simulink model "controller"  (R2023a)
settings: Solver=VariableStepAuto  StartTime=0.0  StopTime=10.0  RelTol=1e-3
undefined symbols (not defined in the file): DiscIntNeverNeededParam
libraries: simulink x1
settings Model: Creator=pengda  LastModifiedBy=pengda

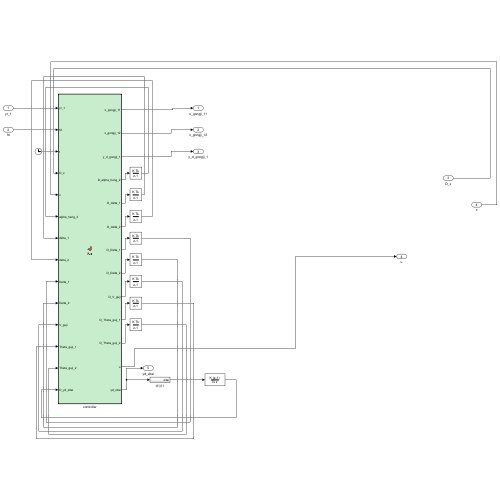
[thumbnail: Simulink's stored preview of the top-level diagram]
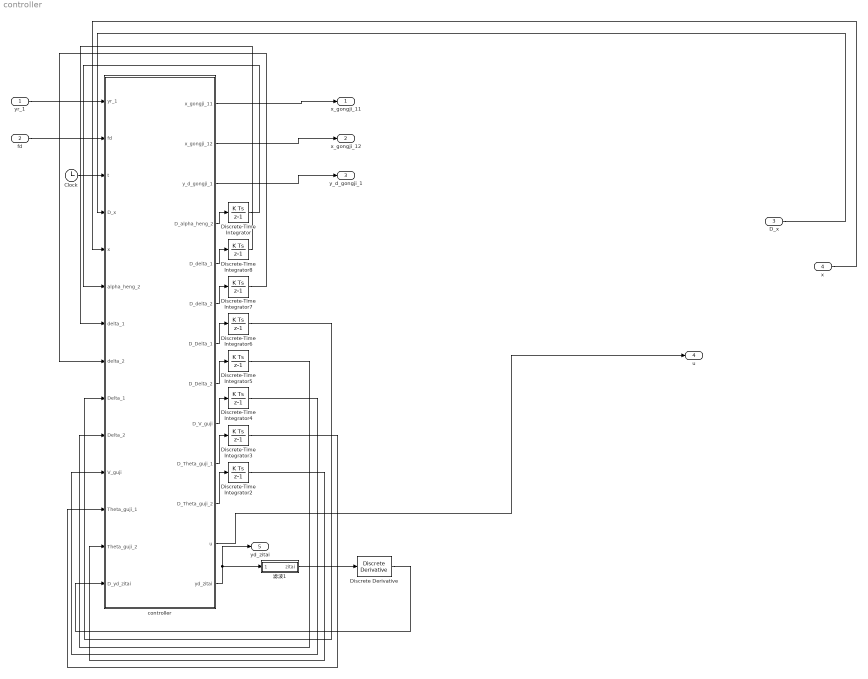
== system controller ==
  yr_1 : Inport
  fd : Inport  Port=2
  D_x : Inport  Port=3
  x : Inport  Port=4
  Clock : Clock
  Discrete Derivative : simulink/Discrete/Discrete Derivative  gainval=1.0  ICPrevScaledInput=0.0  OutMin=[]  OutMax=[]  OutDataType=fixdt(1, 16)  OutScaling=2^-10  DoSatur=off
  Discrete-Time Integrator{,5..8} (5 alike) : DiscreteIntegrator  InitialCondition=[0;0;0;0;0;0]  SampleTime=-1  ICPrevOutput=DiscIntNeverNeededParam  ICPrevScaledInput=DiscIntNeverNeededParam
  Discrete-Time Integrator2 : DiscreteIntegrator  InitialCondition=[1.2;1.2;1.2;0.2;0.2;0.2]  SampleTime=-1  ICPrevOutput=DiscIntNeverNeededParam  ICPrevScaledInput=DiscIntNeverNeededParam
  Discrete-Time Integrator3 : DiscreteIntegrator  InitialCondition=[2.2;2.2;2.2;0;0;0]  SampleTime=-1  ICPrevOutput=DiscIntNeverNeededParam  ICPrevScaledInput=DiscIntNeverNeededParam
  Discrete-Time Integrator4 : DiscreteIntegrator  InitialCondition=[4;4;4;0;0;0]  SampleTime=-1  ICPrevOutput=DiscIntNeverNeededParam  ICPrevScaledInput=DiscIntNeverNeededParam
  controller : MATLAB Function  TreatAsAtomicUnit=on
  滤波1 : Subsystem
  x_gongji_11 : Outport
  x_gongji_12 : Outport  Port=2
  y_d_gongji_1 : Outport  Port=3
  u : Outport  Port=4
  yd_zitai : Outport  Port=5
  wires:
  controller/8(D_Delta_2) -> Discrete-Time Integrator5/1
  controller/1(x_gongji_11) -> x_gongji_11/1
  controller/12(u) -> u/1
  controller/3(y_d_gongji_1) -> y_d_gongji_1/1
  controller/4(D_alpha_heng_2) -> Discrete-Time Integrator/1
  controller/13(yd_zitai) -> yd_zitai/1, 滤波1/1(" ")
  controller/10(D_Theta_guji_1) -> Discrete-Time Integrator3/1
  controller/11(D_Theta_guji_2) -> Discrete-Time Integrator2/1
  滤波1/1(zitai) -> Discrete Derivative/1
  D_x/1 -> controller/4(D_x)
  Discrete-Time Integrator3/1 -> controller/12(Theta_guji_1)
  fd/1 -> controller/2(fd)
  Clock/1 -> controller/3(t)
  controller/5(D_delta_1) -> Discrete-Time Integrator8/1
  yr_1/1 -> controller/1(yr_1)
  Discrete Derivative/1 -> controller/14(D_yd_zitai)
  controller/2(x_gongji_12) -> x_gongji_12/1
  Discrete-Time Integrator8/1 -> controller/7(delta_1)
  Discrete-Time Integrator6/1 -> controller/9(Delta_1)
  controller/6(D_delta_2) -> Discrete-Time Integrator7/1
  Discrete-Time Integrator5/1 -> controller/10(Delta_2)
  controller/9(D_V_guji) -> Discrete-Time Integrator4/1
  Discrete-Time Integrator2/1 -> controller/13(Theta_guji_2)
  Discrete-Time Integrator/1 -> controller/6(alpha_heng_2)
  controller/7(D_Delta_1) -> Discrete-Time Integrator6/1
  Discrete-Time Integrator4/1 -> controller/11(V_guji)
  Discrete-Time Integrator7/1 -> controller/8(delta_2)
  x/1 -> controller/5(x)

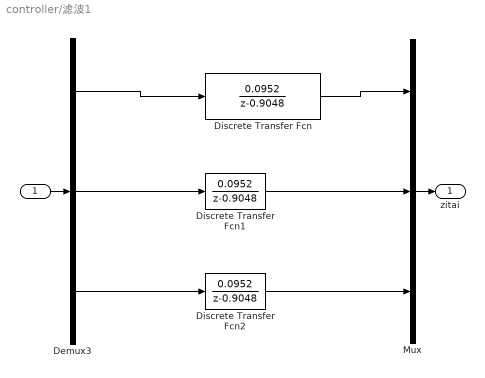
== system controller/滤波1 ==
  " " : Inport
  Demux3 : Demux  Outputs=3
  Discrete Transfer Fcn : DiscreteTransferFcn  Numerator=[0.0952]  Denominator=[1, -0.9048]
  Discrete Transfer Fcn1 : DiscreteTransferFcn  Numerator=[0.0952]  Denominator=[1, -0.9048]
  Discrete Transfer Fcn2 : DiscreteTransferFcn  Numerator=[0.0952]  Denominator=[1, -0.9048]
  Mux : Mux  Inputs=3
  zitai : Outport  VectorParamsAs1DForOutWhenUnconnected=off
  wires:
  Demux3/3 -> Discrete Transfer Fcn2/1
  Discrete Transfer Fcn2/1 -> Mux/3
  Discrete Transfer Fcn/1 -> Mux/1
  Discrete Transfer Fcn1/1 -> Mux/2
  Demux3/1 -> Discrete Transfer Fcn/1
  Demux3/2 -> Discrete Transfer Fcn1/1
  Mux/1 -> zitai/1
  " "/1 -> Demux3/1

== matlab function controller/controller ==
  data: yr_1 input; fd input; t input; D_x input; x input; x_gongji_11 output; x_gongji_12 output; y_d_gongji_1 output; alpha_heng_2 input; delta_1 input; delta_2 input; Delta_1 input; Delta_2 input; V_guji input; Theta_guji_1 input; Theta_guji_2 input; D_alpha_heng_2 output; D_delta_1 output; D_delta_2 output; D_Delta_1 output; D_Delta_2 output; D_V_guji output; D_Theta_guji_1 output; D_Theta_guji_2 output; u output; D_yd_zitai input; yd_zitai output
function [x_gongji_11,x_gongji_12,y_d_gongji_1, D_alpha_heng_2, D_delta_1, D_delta_2, D_Delta_1,D_Delta_2, D_V_guji, D_Theta_guji_1,D_Theta_guji_2, u, yd_zitai]  =   fcn( yr_1, fd, t, D_x, x, alpha_heng_2, delta_1,delta_2, Delta_1,Delta_2, V_guji, Theta_guji_1,Theta_guji_2,D_yd_zitai)
%%
%%%%%%%%%%%%%%%%%%%%%%%%%%%%%%%%%%%%%%%%%%%%%%%%%%%%%%%%%%%%%%%%%%%%%%%%%%%%%%%%%%%%%%%%%%%%%%%%%%%%%%%%%%%%%%%%%%%%%%%%%%%%%
%                                      控制器参数
% % 通信拓步图参数
%   X          Y
 af1 = 1;    %领航者
 af2 = 0;    %2号
 af3 = 0;    %3号
 af4 = 0;    %4号
 af5 = 0;    %5号

%%%%%%%%%%%%%%%%%%%%%%%%%%%%
%%%%%%%%%%%%%%%%%%%%%%%%%
%%
%动力学参数
m = 1.8;
g = 9.81;

fx=0.001;%平移阻力系数
fy=0.001;
fz=0.001;
f_theta=0.15;
f_phi=0.15;
f_psi=0.15;

I_xx = 0.75;      % 四旋翼x轴转动惯量(kg·m^2)
I_yy = 0.75;      % 四旋翼y轴转动惯量(kg·m^2)
I_zz = 1.5;       % 四旋翼z轴转动惯量(kg·m^2)
J_RP = 0.0000616;   % 整个电机转子和螺旋桨绕转轴的总转动惯量(kg·m^2)
d = 0.2;          % 机体中心和任一电机的距离(m)


%执行器故障
rho_1 = 0.8;
rho_2 = 0.8;
rho_3 = 1;
rho_4 = 1;
rho_5 = 1;
rho_6 = 1;

yita_1 = 0.02*cos(0.2*t);
yita_2 = 0.02*cos(0.2*t);
yita_3 = 0;
yita_4 = 0;
yita_5 = 0;
yita_6 = 0;

%滤波器参数  重要<1
epsilon_12=0.01;
epsilon_22=0.01;
epsilon_32=0.01;
epsilon_42=0.03;
epsilon_52=0.05;
epsilon_62=0.08;

%控制器参数
T=3;
zeta=1;

c=70;
l=0.03;%0.03

t_1=12;
t_2=11;
t_3=11;
t_4=2;
t_5=2;
t_6=2;

k_11=60;%重要
k_21=40;
k_31=50;
k_41=40;
k_51=40;
k_61=40;

k_12=60;%重要
k_22=40;
k_32=50;
k_42=40;
k_52=40;
k_62=40;

l_11=1.5;
l_21=1.5;
l_31=1.5;
l_41=1.5;
l_51=1.5;
l_61=1.5;

l_12=1;
l_22=1;
l_32=1;
l_42=1;
l_52=1;
l_62=1;

sigma_11=32;
sigma_21=48;
sigma_31=45;
sigma_41=32;
sigma_51=37;
sigma_61=36;

sigma_12=3.6;%重要
sigma_22=3.5;
sigma_32=3.2;
sigma_42=2.7;
sigma_52=2.8;
sigma_62=3.1;

%
p=2;

E=10;

g_1=8;%重要
g_2=8;
g_3=8;
g_4=10;
g_5=10;
g_6=10;



%
D_X=D_x(1);
D_Y=D_x(2);
D_Z=D_x(3);
D_theta=D_x(4);
D_phi=D_x(5);
D_psi=D_x(6);

X=x(1);
Y=x(2);
Z=x(3);
theta=x(4);
phi=x(5);
psi=x(6);

yd_1=yr_1(1);
yd_2=yr_1(2);
yd_3=yr_1(3);

fd_1=fd(1);
fd_2=fd(2);
fd_3=fd(3);

fd_4=D_yd_zitai(1);
fd_5=D_yd_zitai(2);
fd_6=D_yd_zitai(3);

alpha_heng_12=alpha_heng_2(1);
alpha_heng_22=alpha_heng_2(2);
alpha_heng_32=alpha_heng_2(3);
alpha_heng_42=alpha_heng_2(4);
alpha_heng_52=alpha_heng_2(5);
alpha_heng_62=alpha_heng_2(6);

delta_11=delta_1(1);
delta_21=delta_1(2);
delta_31=delta_1(3);
delta_41=delta_1(4);
delta_51=delta_1(5);
delta_61=delta_1(6);

delta_12=delta_2(1);
delta_22=delta_2(2);
delta_32=delta_2(3);
delta_42=delta_2(4);
delta_52=delta_2(5);
delta_62=delta_2(6);

Delta_11=Delta_1(1);
Delta_21=Delta_1(2);
Delta_31=Delta_1(3);
Delta_41=Delta_1(4);
Delta_51=Delta_1(5);
Delta_61=Delta_1(6);

Delta_12=Delta_2(1);
Delta_22=Delta_2(2);
Delta_32=Delta_2(3);
Delta_42=Delta_2(4);
Delta_52=Delta_2(5);
Delta_62=Delta_2(6);

V_guji_1=V_guji(1);
V_guji_2=V_guji(2);
V_guji_3=V_guji(3);
V_guji_4=V_guji(4);
V_guji_5=V_guji(5);
V_guji_6=V_guji(6);

Theta_guji_11=Theta_guji_1(1);
Theta_guji_21=Theta_guji_1(2);
Theta_guji_31=Theta_guji_1(3);
Theta_guji_41=Theta_guji_1(4);
Theta_guji_51=Theta_guji_1(5);
Theta_guji_61=Theta_guji_1(6);

Theta_guji_12=Theta_guji_2(1);
Theta_guji_22=Theta_guji_2(2);
Theta_guji_32=Theta_guji_2(3);
Theta_guji_42=Theta_guji_2(4);
Theta_guji_52=Theta_guji_2(5);
Theta_guji_62=Theta_guji_2(6);


%%%%%%%%%%%%%%%%%%%%%%%%%%%%%%%%%%%%%%%%%%%%%%%%%%%%%%%%%%%%%%%%%%%%%%%%%%%%%%%%%%%%%%%%%%%%%%%%%%%%%%%%%%% 编队
%%%%%%%%%%%%%%%%%%%%%%%%%%%%%%%%%%%%%%%%%%%%%%%%%%%%%%%%%%%%%%%%%%%%%%%%%%%%%%%%%%%%%%%%%%%%%%%%%%%%%%%%%%%
%% 偏移量
% 偏差
y_offest_1 = -1;
y_offest_2 = -1;
y_offest_3 = 0;

x_offest_112 = 0;%对y_offest_1求导
x_offest_122 = 0;
x_offest_132 = 0;


% 编队信息
y_d_1 = yd_1 + y_offest_1;
y_d_2 = yd_2 + y_offest_2;
y_d_3 = yd_3 + y_offest_3;

%%%%%%%%%%%%%%%%%%%%%%%%%%%%%%%%%%%%%%%%%%%%%%%%%%%%%%%%%%%%%%%%%%%%%%%%%%%%%%%%%%%%%%%%%%%%%%%%%%%%%%%%%%% 欺骗攻击 
%%%%%%%%%%%%%%%%%%%%%%%%%%%%%%%%%%%%%%%%%%%%%%%%%%%%%%%%%%%%%%%%%%%%%%%%%%%%%%%%%%%%%%%%%%%%%%%%%%%%%%%%%%%
%% 欺骗攻击

if t<10
    o = 0;
else
    o = -0.01*cos(0.25*t);%更改后导数D_lambda更改
end

% o_1 = -0.2*cos(0.25*t);o_2 = -0.2*cos(0.25*t);o_3 = -0.2*cos(0.25*t);
% o_4 = -0.2*cos(0.25*t);o_5 = -0.2*cos(0.25*t);o_6 = -0.2*cos(0.25*t);

lambda = 1 + o;

if t<10
    D_lambda = 0; 
else
    D_lambda = 0.01*0.25*sin(0.25*t); 
end


% 实际状态一阶
x_gongji_111 = lambda * X ;
x_gongji_121 = lambda * Y ;
x_gongji_131 = lambda * Z ;
x_gongji_141 = lambda * theta ;
x_gongji_151 = lambda * phi ;
x_gongji_161 = lambda * psi ;

% 实际状态二阶
x_gongji_112 = lambda * D_X ;
x_gongji_122 = lambda * D_Y ;
x_gongji_132 = lambda * D_Z ;
x_gongji_142 = lambda * D_theta ;
x_gongji_152 = lambda * D_phi ;
x_gongji_162 = lambda * D_psi ;

% 期望状态
yd_gongji_1 = lambda * yd_1 ;
yd_gongji_2 = lambda * yd_2 ;
yd_gongji_3 = lambda * yd_3 ;


% 编队信息-攻击
y_d_gongji_11 = yd_gongji_1 + y_offest_1;
y_d_gongji_12 = yd_gongji_2 + y_offest_2;
y_d_gongji_13 = yd_gongji_3 + y_offest_3;


%%%%%%%%%%%%%%%%%%%%%%%%%%%%%%%%%%%%%%%%%%%%%%%%%%%%%%%%%%%%%%%%%%%%%%%%%%%%%%%%%%%%%%%%%%%%%%%%%%%%%%%%%%%  动力学模型 位置
%%%%%%%%%%%%%%%%%%%%%%%%%%%%%%%%%%%%%%%%%%%%%%%%%%%%%%%%%%%%%%%%%%%%%%%%%%%%%%%%%%%%%%%%%%%%%%%%%%%%%%%%%%%
%% 动力学模型  位置
%跟随者
F1=-fx*D_X/m ;
F2=-fy*D_Y/m ;
F3=-g-fz*D_Z/m ;

d_x=0.2*sin(t);d_y=0.0001*cos(t);d_z=0.15;
N1=d_x/m;
N2=d_y/m;
N3=d_z/m;

%%%%%%%%%%%%%%%%%%%%%%%%%%%%%%%%%%%%%%%%%%%%%%%%%%%%%%%%%%%%%%%%%%%%%%%%%%%%%%%%%%%%%%%%%%%%%%%%%%%%%%%%%%%  位置控制器
%%%%%%%%%%%%%%%%%%%%%%%%%%%%%%%%%%%%%%%%%%%%%%%%%%%%%%%%%%%%%%%%%%%%%%%%%%%%%%%%%%%%%%%%%%%%%%%%%%%%%%%%%%%
%% 一阶控制器

y_gongji_11 = x_gongji_111;  % y_gongji_i,m ; x_gongji_i,m,s
y_gongji_12 = x_gongji_121;
y_gongji_13 = x_gongji_131;

z_11 = 0 + g_1*(y_gongji_11-y_d_gongji_11);
z_21 = 0 + g_2*(y_gongji_12-y_d_gongji_12);
z_31 = 0 + g_3*(y_gongji_13-y_d_gongji_13);


if t >= 0 && t <= T 
    v = (1/((t+0.01)^2) - 1/(T^2))^(2*p) + zeta;  % eps是MATLAB内置极小值（~2.2e-16）
    D_v = -4*p * (1/((t+0.01)^2) - 1/(T^2))^(2*p - 1) / (t + 0.01)^3;
    % D_v=-(4*p/t^3)*(1/((t+0.01)^2) - 1/T^2)^(2*p-1);
else
    v = zeta;
    D_v = 0;
end


beta_1 = c*(v^2-z_11^2);    % beta_m 
beta_2 = c*(v^2-z_21^2); 
beta_3 = c*(v^2-z_31^2); 

if beta_1 > 0 && beta_1 <= l  
    h_1 = 1-(beta_1/l - 1)^(2*p);    % h_m 
elseif beta_1>l
    h_1=1;
else
    h_1=1;
end

if beta_2 > 0 && beta_2 <= l  
    h_2 = 1-(beta_2/l - 1)^(2*p);    % h_m 
elseif beta_2>l
    h_2=1;
else
    h_2=1;
end

if beta_3 > 0 && beta_3 <= l  
    h_3 = 1-(beta_3/l - 1)^(2*p);    % h_m 
elseif beta_3>l
    h_3=1;
else
    h_3=1;
end

H_11 = z_11/h_1;    % H_m,1
H_21 = z_21/h_2;
H_31 = z_31/h_3;


xi_11 = H_11;
xi_21 = H_21;
xi_31 = H_31;


if beta_1 > 0 && beta_1 <= l  
    mu_1 = 1/h_1 - (4*c*p/(l*h_1^2))*((beta_1/l - 1)^(2*p-1))*z_11^2;    % mu_m 
elseif beta_1>l
    mu_1=1;
else
    mu_1=1;
end

if beta_2 > 0 && beta_2 <= l  
    mu_2 = 1/h_2 - (4*c*p/(l*h_2^2))*((beta_2/l - 1)^(2*p-1))*z_21^2;    % mu_m 
elseif beta_2>l
    mu_2=1;
else
    mu_2=1;
end

if beta_3 > 0 && beta_3 <= l  
    mu_3 = 1/h_3 - (4*c*p/(l*h_3^2))*((beta_3/l - 1)^(2*p-1))*z_31^2;    % mu_m 
elseif beta_3>l
    mu_3=1;
else
    mu_3=1;
end

d_i= af2 + af3 + af4 + af5;

tau_1 = d_i + g_1;
tau_2 = d_i + g_2;
tau_3 = d_i + g_3;


B_1 = D_lambda*(lambda\tau_1)*x_gongji_111 - 0 - D_lambda*(lambda\g_1)*yd_gongji_1 - lambda*g_1*fd_1 - 0 + 0;
B_2 = D_lambda*(lambda\tau_2)*x_gongji_121 - 0 - D_lambda*(lambda\g_2)*yd_gongji_2 - lambda*g_2*fd_2 - 0 + 0;
B_3 = D_lambda*(lambda\tau_3)*x_gongji_131 - 0 - D_lambda*(lambda\g_3)*yd_gongji_3 - lambda*g_3*fd_3 - 0 + 0;




if beta_1 > 0 && beta_1 <= l  
    v_1 = (4*c*p/(l*h_1^2))*((beta_1/l - 1)^(2*p-1))*v*D_v*z_11;    % v_m 
elseif beta_1>l
    v_1=0;
else
    v_1=0;
end

if beta_2 > 0 && beta_2 <= l  
    v_2 = (4*c*p/(l*h_2^2))*((beta_2/l - 1)^(2*p-1))*v*D_v*z_21;    % v_m 
elseif beta_2>l
    v_2=0;
else
    v_2=0;
end

if beta_3 > 0 && beta_3 <= l  
    v_3 = (4*c*p/(l*h_3^2))*((beta_3/l - 1)^(2*p-1))*v*D_v*z_31;    % v_m 
elseif beta_3>l
    v_3=0;
else
    v_3=0;
end


alpha_11 = (-k_11*xi_11 - (Delta_11*mu_1^2*(E+1))/(4*sqrt(Delta_11^2*mu_1^2+sigma_11^2)) - Delta_11*mu_1^2*Theta_guji_11/sqrt(Delta_11^2*mu_1^2+sigma_11^2) - v_1 - (l_11*delta_11)/sqrt(delta_11^2+sigma_11^2))/(mu_1*tau_1);
alpha_21 = (-k_21*xi_21 - (Delta_21*mu_2^2*(E+1))/(4*sqrt(Delta_21^2*mu_2^2+sigma_21^2)) - Delta_21*mu_2^2*Theta_guji_21/sqrt(Delta_21^2*mu_2^2+sigma_21^2) - v_2 - (l_21*delta_21)/sqrt(delta_21^2+sigma_21^2))/(mu_2*tau_2);
alpha_31 = (-k_31*xi_31 - (Delta_31*mu_3^2*(E+1))/(4*sqrt(Delta_31^2*mu_3^2+sigma_31^2)) - Delta_31*mu_3^2*Theta_guji_31/sqrt(Delta_31^2*mu_3^2+sigma_31^2) - v_3 - (l_31*delta_31)/sqrt(delta_31^2+sigma_31^2))/(mu_3*tau_3);


D_Theta_guji_11 = Delta_11^2*mu_1^2/sqrt(Delta_11^2*mu_1^2+sigma_11^2) - sigma_11*Theta_guji_11;
D_Theta_guji_21 = Delta_21^2*mu_2^2/sqrt(Delta_21^2*mu_2^2+sigma_21^2) - sigma_21*Theta_guji_21;
D_Theta_guji_31 = Delta_31^2*mu_3^2/sqrt(Delta_31^2*mu_3^2+sigma_31^2) - sigma_31*Theta_guji_31;


D_delta_11 = -k_11*delta_11 + mu_1*tau_1*(alpha_heng_12-alpha_11) + mu_1*tau_1*delta_12 - (l_11*delta_11)/sqrt(delta_11^2+sigma_11^2);
D_delta_21 = -k_21*delta_21 + mu_2*tau_2*(alpha_heng_22-alpha_21) + mu_2*tau_2*delta_22 - (l_21*delta_21)/sqrt(delta_21^2+sigma_21^2);
D_delta_31 = -k_31*delta_31 + mu_3*tau_3*(alpha_heng_32-alpha_31) + mu_3*tau_3*delta_32 - (l_31*delta_31)/sqrt(delta_31^2+sigma_31^2);


D_Delta_11 = mu_1*tau_1*(Delta_12+alpha_11-x_offest_112) + mu_1*B_1 + v_1 + k_11*delta_11 + (l_11*delta_11)/sqrt(delta_11^2+sigma_11^2);
D_Delta_21 = mu_2*tau_2*(Delta_22+alpha_21-x_offest_122) + mu_2*B_2 + v_2 + k_21*delta_21 + (l_21*delta_21)/sqrt(delta_21^2+sigma_21^2);
D_Delta_31 = mu_3*tau_3*(Delta_32+alpha_31-x_offest_132) + mu_3*B_3 + v_3 + k_31*delta_31 + (l_31*delta_31)/sqrt(delta_31^2+sigma_31^2);



%% 二阶控制器


xi_12 = x_gongji_112-alpha_heng_12;
xi_22 = x_gongji_122-alpha_heng_22;
xi_32 = x_gongji_132-alpha_heng_32;


D_alpha_heng_12=(alpha_11-alpha_heng_12)/epsilon_12;
D_alpha_heng_22=(alpha_21-alpha_heng_22)/epsilon_22;
D_alpha_heng_32=(alpha_31-alpha_heng_32)/epsilon_32;


D_delta_12 = -k_12*delta_12 - (l_12*delta_12)/sqrt(delta_12^2+sigma_12^2);
D_delta_22 = -k_22*delta_22 - (l_22*delta_22)/sqrt(delta_22^2+sigma_22^2);
D_delta_32 = -k_32*delta_32 - (l_32*delta_32)/sqrt(delta_32^2+sigma_32^2);


D_Theta_guji_12 = Delta_12^2/sqrt(Delta_12^2+sigma_12^2) - sigma_12*Theta_guji_12;
D_Theta_guji_22 = Delta_22^2/sqrt(Delta_22^2+sigma_22^2) - sigma_22*Theta_guji_22;
D_Theta_guji_32 = Delta_32^2/sqrt(Delta_32^2+sigma_32^2) - sigma_32*Theta_guji_32;


pi_1 = k_12*xi_12 + (Delta_12*(E+1))/(4*sqrt(Delta_12^2+sigma_12^2)) + (Delta_12*Theta_guji_12)/sqrt(Delta_12^2+sigma_12^2) - D_alpha_heng_12 + (l_12*delta_12)/sqrt(delta_12^2+sigma_12^2) + Delta_11;
pi_2 = k_22*xi_22 + (Delta_22*(E+1))/(4*sqrt(Delta_22^2+sigma_22^2)) + (Delta_22*Theta_guji_22)/sqrt(Delta_22^2+sigma_22^2) - D_alpha_heng_22 + (l_22*delta_22)/sqrt(delta_22^2+sigma_22^2) + Delta_21;
pi_3 = k_32*xi_32 + (Delta_32*(E+1))/(4*sqrt(Delta_32^2+sigma_32^2)) + (Delta_32*Theta_guji_32)/sqrt(Delta_32^2+sigma_32^2) - D_alpha_heng_32 + (l_32*delta_32)/sqrt(delta_32^2+sigma_32^2) + Delta_31;


D_V_guji_1 = Delta_12*pi_1 - sigma_12*V_guji_1;
D_V_guji_2 = Delta_22*pi_2 - sigma_22*V_guji_2;
D_V_guji_3 = Delta_32*pi_3 - sigma_32*V_guji_3;


% u1 = -(Delta_12*V_guji_1^2*pi_1^2)/(C1*sqrt(Delta_12^2*V_guji_1^2*pi_1^2+t_1^2));
u1 = -(Delta_12*V_guji_1^2*pi_1^2)/(sqrt(Delta_12^2*V_guji_1^2*pi_1^2+t_1^2));
u2 = -(Delta_22*V_guji_2^2*pi_2^2)/(sqrt(Delta_22^2*V_guji_2^2*pi_2^2+t_2^2));
u3 = -(Delta_32*V_guji_3^2*pi_3^2)/(sqrt(Delta_32^2*V_guji_3^2*pi_3^2+t_3^2));


D_Delta_12 = D_lambda*(lambda\x_gongji_112) + lambda*rho_1*u1 - D_alpha_heng_12 + lambda*yita_1 + lambda*F1 + lambda*N1 + k_12*delta_12 + (l_12*delta_12)/sqrt(delta_12^2+sigma_12^2);
D_Delta_22 = D_lambda*(lambda\x_gongji_122) + lambda*rho_2*u2 - D_alpha_heng_22 + lambda*yita_2 + lambda*F2 + lambda*N2 + k_22*delta_22 + (l_22*delta_22)/sqrt(delta_22^2+sigma_22^2);
D_Delta_32 = D_lambda*(lambda\x_gongji_132) + lambda*rho_3*u3 - D_alpha_heng_32 + lambda*yita_3 + lambda*F3 + lambda*N3 + k_32*delta_32 + (l_32*delta_32)/sqrt(delta_32^2+sigma_32^2);


%%%%%%%%%%%%%%%%%%%%%%%%%%%%%%%%%%%%%%%%%%%%%%%%%%%%%%%%%%%%%%%%%%%%%%%%%%%%%%%%%%%%%%%%%%%%%%%%%%%%%%%%%%%  姿态动力学模型
%%%%%%%%%%%%%%%%%%%%%%%%%%%%%%%%%%%%%%%%%%%%%%%%%%%%%%%%%%%%%%%%%%%%%%%%%%%%%%%%%%%%%%%%%%%%%%%%%%%%%%%%%%%
%% 动力学模型
%跟随者 姿态
c_T = 120;    % 螺旋桨拉力系数
c_M = 0.033;  % 螺旋桨力矩系数
F = m *((u1)^2 + (u2)^2 + (u3)^2)^0.5;

w1= (abs(F/c_T + (2)^0.5*u1/(d*c_T) + (2)^0.5*u2/(d*c_T) + u3/(c_T*c_M))/4)^0.5;
w2= (abs(F/c_T - (2)^0.5*u1/(d*c_T) + (2)^0.5*u2/(d*c_T) - u3/(c_T*c_M))/4)^0.5;
w3= (abs(F/c_T - (2)^0.5*u1/(d*c_T) - (2)^0.5*u2/(d*c_T) + u3/(c_T*c_M))/4)^0.5;
w4= (abs(F/c_T + (2)^0.5*u1/(d*c_T) - (2)^0.5*u2/(d*c_T) - u3/(c_T*c_M))/4)^0.5;

Omega=-w1+w2-w3+w4;

a1=(I_zz-I_xx)/I_yy; a2=J_RP/I_yy; a3=f_theta/I_yy;
a4=(I_yy-I_zz)/I_xx; a5=J_RP/I_xx; a6=f_phi/I_xx;
a7=(I_xx-I_yy)/I_zz;a8=f_psi/I_zz;

F4=a1*D_phi*D_psi-a2*D_phi*Omega-a3*D_theta;
F5=a4*D_theta*D_psi-a5*D_theta*Omega-a6*D_phi;
F6=a7*D_theta*D_phi-a8*D_psi;

% d_x=0.2*sin(t);d_y=0.05*cos(t)+0.001sin(Y);d_z=0.15;
% d_theta=0.05*sin(t);d_phi=0.01;d_psi=0.02*cos(5*theta);

d_theta=0.05*sin(t); d_phi=0.01; d_psi=0.02*cos(5*theta);

N4 = d_theta/I_yy;
N5 = d_phi/I_xx;
N6 = d_psi/I_zz;
%%%%%%%%%%%%%%%%%%%%%%%%%%%%%%%%%%%%%%%%%%%%%%%%%%%%%%%%%%%%%%%%%%%%%%%%%%%%%%%%%%%%%%%%%%%%%%%%%%%%%%%%%%%  姿态控制器
%%%%%%%%%%%%%%%%%%%%%%%%%%%%%%%%%%%%%%%%%%%%%%%%%%%%%%%%%%%%%%%%%%%%%%%%%%%%%%%%%%%%%%%%%%%%%%%%%%%%%%%%%%%
%%%%%%%%%%%%%%%%%%%%%%%%%%%%%%%%%%%%%%%%%%%%%%%%%%%%%%%%%%%%%%%%%%%%%%%%%%%

psi_d=1+0.1*sin(t);

yd_4=asin( (sin(psi_d)*u1 - cos(psi_d)*u2) / sqrt(u1^2 + u2^2 + u3^2 + 1e-6) );
yd_5=atan( (cos(psi_d)*u1 + sin(psi_d)*u2) / (u3 + 1e-6));
yd_6=psi_d;



%% 欺骗攻击
% 期望状态 
yd_gongji_4 = lambda * yd_4 ;
yd_gongji_5 = lambda * yd_5 ;
yd_gongji_6 = lambda * yd_6 ;


%% 一阶控制器

y_gongji_14 = x_gongji_141;  % y_gongji_i,m ; x_gongji_m,s
y_gongji_15 = x_gongji_151;
y_gongji_16 = x_gongji_161;

z_41 =  g_4*(y_gongji_14-yd_gongji_4);   % offest_gongji_m
z_51 =  g_5*(y_gongji_15-yd_gongji_5);
z_61 =  g_6*(y_gongji_16-yd_gongji_6);


beta_4 = c*(v^2-z_41^2);    % beta_m 
beta_5 = c*(v^2-z_51^2); 
beta_6 = c*(v^2-z_61^2);


if beta_4 > 0 && beta_4 <= l  
    h_4 = 1-(beta_4/l - 1)^(2*p);    % h_m 
elseif beta_4>l
    h_4=1;
else
    h_4=1;
end

if beta_5 > 0 && beta_5 <= l  
    h_5 = 1-(beta_5/l - 1)^(2*p);    % h_m 
elseif beta_5>l
    h_5=1;
else
    h_5=1;
end

if beta_6 > 0 && beta_6 <= l  
    h_6 = 1-(beta_6/l - 1)^(2*p);    % h_m 
elseif beta_6>l
    h_6=1;
else
    h_6=1;
end


H_41 = z_41/h_4;    % H_m,1
H_51 = z_51/h_5;
H_61 = z_61/h_6;


xi_41 = H_41;
xi_51 = H_51;
xi_61 = H_61;


if beta_4 > 0 && beta_4 <= l  
    mu_4 = 1/h_4 - (4*c*p/(l*h_4^2))*((beta_4/l - 1)^(2*p-1))*z_41^2;    % mu_m 
elseif beta_4>l
    mu_4=1;
else
    mu_4=1;
end

if beta_5 > 0 && beta_5 <= l  
    mu_5 = 1/h_5 - (4*c*p/(l*h_5^2))*((beta_5/l - 1)^(2*p-1))*z_51^2;    % mu_m 
elseif beta_5>l
    mu_5=1;
else
    mu_5=1;
end

if beta_6 > 0 && beta_6 <= l  
    mu_6 = 1/h_6 - (4*c*p/(l*h_6^2))*((beta_6/l - 1)^(2*p-1))*z_61^2;    % mu_m 
elseif beta_6>l
    mu_6=1;
else
    mu_6=1;
end


B_4 = D_lambda*(lambda\g_4)*x_gongji_141 - D_lambda*(lambda\g_4)*yd_gongji_4 - lambda*g_4*fd_4;
B_5 = D_lambda*(lambda\g_5)*x_gongji_151 - D_lambda*(lambda\g_5)*yd_gongji_5 - lambda*g_5*fd_5;
B_6 = D_lambda*(lambda\g_6)*x_gongji_161 - D_lambda*(lambda\g_6)*yd_gongji_6 - lambda*g_6*fd_6;


if beta_4 > 0 && beta_4 <= l  
    v_4 = (4*c*p/(l*h_4^2))*((beta_4/l - 1)^(2*p-1))*v*D_v*z_41;    % v_m 
elseif beta_4>l
    v_4=0;
else
    v_4=0;
end

if beta_5 > 0 && beta_5 <= l  
    v_5 = (4*c*p/(l*h_5^2))*((beta_5/l - 1)^(2*p-1))*v*D_v*z_51;    % v_m 
elseif beta_5>l
    v_5=0;
else
    v_5=0;
end

if beta_6 > 0 && beta_6 <= l  
    v_6 = (4*c*p/(l*h_6^2))*((beta_6/l - 1)^(2*p-1))*v*D_v*z_61;    % v_m 
elseif beta_6>l
    v_6=0;
else
    v_6=0;
end


alpha_41 = (-k_41*xi_41 - (Delta_41*mu_4^2*(E+1))/(4*sqrt(Delta_41^2*mu_4^2+sigma_41^2)) - Delta_41*mu_4^2*Theta_guji_41/sqrt(Delta_41^2*mu_4^2+sigma_41^2) - v_4 - (l_41*delta_41)/sqrt(delta_41^2+sigma_41^2))/(mu_4*g_4);
alpha_51 = (-k_51*xi_51 - (Delta_51*mu_5^2*(E+1))/(4*sqrt(Delta_51^2*mu_5^2+sigma_51^2)) - Delta_51*mu_5^2*Theta_guji_51/sqrt(Delta_51^2*mu_5^2+sigma_51^2) - v_5 - (l_51*delta_51)/sqrt(delta_51^2+sigma_51^2))/(mu_5*g_5);
alpha_61 = (-k_61*xi_61 - (Delta_61*mu_6^2*(E+1))/(4*sqrt(Delta_61^2*mu_6^2+sigma_61^2)) - Delta_61*mu_6^2*Theta_guji_61/sqrt(Delta_61^2*mu_6^2+sigma_61^2) - v_6 - (l_61*delta_61)/sqrt(delta_61^2+sigma_61^2))/(mu_6*g_6);


D_Theta_guji_41 = Delta_41^2*mu_4^2/sqrt(Delta_41^2*mu_4^2+sigma_41^2) - sigma_41*Theta_guji_41;
D_Theta_guji_51 = Delta_51^2*mu_5^2/sqrt(Delta_51^2*mu_5^2+sigma_51^2) - sigma_51*Theta_guji_51;
D_Theta_guji_61 = Delta_61^2*mu_6^2/sqrt(Delta_61^2*mu_6^2+sigma_61^2) - sigma_61*Theta_guji_61;


D_delta_41 = -k_41*delta_41 + mu_4*g_4*(alpha_heng_42-alpha_41) + mu_4*g_4*delta_42 - (l_41*delta_41)/sqrt(delta_41^2+sigma_41^2);
D_delta_51 = -k_51*delta_51 + mu_5*g_5*(alpha_heng_52-alpha_51) + mu_5*g_5*delta_52 - (l_51*delta_51)/sqrt(delta_51^2+sigma_51^2);
D_delta_61 = -k_61*delta_61 + mu_6*g_6*(alpha_heng_62-alpha_61) + mu_6*g_6*delta_62 - (l_61*delta_61)/sqrt(delta_61^2+sigma_61^2);


D_Delta_41 = mu_4*g_4*(Delta_42+alpha_41) + mu_4*B_4 + v_4 + k_41*delta_41 + (l_41*delta_41)/sqrt(delta_41^2+sigma_41^2);
D_Delta_51 = mu_5*g_5*(Delta_52+alpha_51) + mu_5*B_5 + v_5 + k_51*delta_51 + (l_51*delta_51)/sqrt(delta_51^2+sigma_51^2);
D_Delta_61 = mu_6*g_6*(Delta_62+alpha_61) + mu_6*B_6 + v_6 + k_61*delta_61 + (l_61*delta_61)/sqrt(delta_61^2+sigma_61^2);


%% 二阶控制器


xi_42 = x_gongji_142-alpha_heng_42;
xi_52 = x_gongji_152-alpha_heng_52;
xi_62 = x_gongji_162-alpha_heng_62;

D_alpha_heng_42=(alpha_41-alpha_heng_42)/epsilon_42;
D_alpha_heng_52=(alpha_51-alpha_heng_52)/epsilon_52;
D_alpha_heng_62=(alpha_61-alpha_heng_62)/epsilon_62;

D_delta_42 = -k_42*delta_42 - (l_42*delta_42)/sqrt(delta_42^2+sigma_42^2);
D_delta_52 = -k_52*delta_52 - (l_52*delta_52)/sqrt(delta_52^2+sigma_52^2);
D_delta_62 = -k_62*delta_62 - (l_62*delta_62)/sqrt(delta_62^2+sigma_62^2);

D_Theta_guji_42 = Delta_42^2/sqrt(Delta_42^2+sigma_42^2) - sigma_42*Theta_guji_42;
D_Theta_guji_52 = Delta_52^2/sqrt(Delta_52^2+sigma_52^2) - sigma_52*Theta_guji_52;
D_Theta_guji_62 = Delta_62^2/sqrt(Delta_62^2+sigma_62^2) - sigma_62*Theta_guji_62;

pi_4 = k_42*xi_42 + (Delta_42*(E+1))/(4*sqrt(Delta_42^2+sigma_42^2)) + (Delta_42*Theta_guji_42)/sqrt(Delta_42^2+sigma_42^2) - D_alpha_heng_42 + (l_42*delta_42)/sqrt(delta_42^2+sigma_42^2) + Delta_41;
pi_5 = k_52*xi_52 + (Delta_52*(E+1))/(4*sqrt(Delta_52^2+sigma_52^2)) + (Delta_52*Theta_guji_52)/sqrt(Delta_52^2+sigma_52^2) - D_alpha_heng_52 + (l_52*delta_52)/sqrt(delta_52^2+sigma_52^2) + Delta_51;
pi_6 = k_62*xi_62 + (Delta_62*(E+1))/(4*sqrt(Delta_62^2+sigma_62^2)) + (Delta_62*Theta_guji_62)/sqrt(Delta_62^2+sigma_62^2) - D_alpha_heng_62 + (l_62*delta_62)/sqrt(delta_62^2+sigma_62^2) + Delta_61;

D_V_guji_4 = Delta_42*pi_4 - sigma_42*V_guji_4;
D_V_guji_5 = Delta_52*pi_5 - sigma_52*V_guji_5;
D_V_guji_6 = Delta_62*pi_6 - sigma_62*V_guji_6;

u4 = -(Delta_42*V_guji_4^2*pi_4^2)/(sqrt(Delta_42^2*V_guji_4^2*pi_4^2+t_4^2));
u5 = -(Delta_52*V_guji_5^2*pi_5^2)/(sqrt(Delta_52^2*V_guji_5^2*pi_5^2+t_5^2));
u6 = -(Delta_62*V_guji_6^2*pi_6^2)/(sqrt(Delta_62^2*V_guji_6^2*pi_6^2+t_6^2));

D_Delta_42 = D_lambda*(lambda\x_gongji_142) + lambda*rho_4*u4 - D_alpha_heng_42 + lambda*yita_4 + lambda*F4 + lambda*N4 + k_42*delta_42 + (l_42*delta_42)/sqrt(delta_42^2+sigma_42^2);
D_Delta_52 = D_lambda*(lambda\x_gongji_152) + lambda*rho_5*u5 - D_alpha_heng_52 + lambda*yita_5 + lambda*F5 + lambda*N5 + k_52*delta_52 + (l_52*delta_52)/sqrt(delta_52^2+sigma_52^2);
D_Delta_62 = D_lambda*(lambda\x_gongji_162) + lambda*rho_6*u6 - D_alpha_heng_62 + lambda*yita_6 + lambda*F6 + lambda*N6 + k_62*delta_62 + (l_62*delta_62)/sqrt(delta_62^2+sigma_62^2);
% D_Delta_42 = 0;
% D_Delta_52 = 0;
% D_Delta_62 = 0;



%%%%%%%%%%%%%%%%%%%%%%%%%%%%%%%%%%%%%%%%%%%%%%%%%%%%%%%%%%%%%%%%%%%%%%%%%%%%%%%%%%%%%%%%%%%%%%%%%%%%%%%%%%%%%%%%%%%%%%%%%%%%%%%%%%%%%%%%%%%%%%%%%%%%
%%%%%%%%%%%%%%%%%%%%%%%%%%%%%%%%%%%%%%%%%%%%%%%%%%%%%%%%%%%%%%%%%%%%%%%%%%%%%%%%%%%%%%%%%%%%%%%%%%%%%%%%%%%%%%%%%%%%%%%%%%%%%%%%%%%%%%%%%%%%%%%%%%%%
x_gongji_11=[x_gongji_111;x_gongji_121;x_gongji_131];
x_gongji_12=[x_gongji_112;x_gongji_122;x_gongji_132];
y_d_gongji_1=[y_d_gongji_11;y_d_gongji_12;y_d_gongji_13];

yd_zitai=[yd_4;yd_5;yd_6];

D_alpha_heng_2=[D_alpha_heng_12;D_alpha_heng_22;D_alpha_heng_32;D_alpha_heng_42;D_alpha_heng_52;D_alpha_heng_62];

D_delta_1=[D_delta_11;D_delta_21;D_delta_31;D_delta_41;D_delta_51;D_delta_61];
D_delta_2=[D_delta_12;D_delta_22;D_delta_32;D_delta_42;D_delta_52;D_delta_62];

D_Delta_1=[D_Delta_11;D_Delta_21;D_Delta_31;D_Delta_41;D_Delta_51;D_Delta_61];
D_Delta_2=[D_Delta_12;D_Delta_22;D_Delta_32;D_Delta_42;D_Delta_52;D_Delta_62];

D_V_guji=[D_V_guji_1;D_V_guji_2;D_V_guji_3;D_V_guji_4;D_V_guji_5;D_V_guji_6];

D_Theta_guji_1=[D_Theta_guji_11;D_Theta_guji_21;D_Theta_guji_31;D_Theta_guji_41;D_Theta_guji_51;D_Theta_guji_61];
D_Theta_guji_2=[D_Theta_guji_12;D_Theta_guji_22;D_Theta_guji_32;D_Theta_guji_42;D_Theta_guji_52;D_Theta_guji_62];

u=[u1;u2;u3;u4;u5;u6];
